simulink model "stpa_brake_manage_loss"  (R2022a)
settings: Solver=VariableStepAuto  StartTime=0.0  StopTime=10.0  RelTol=1e-3
settings Model: Creator=E403510  LastModifiedBy=ayj
settings SolverCC: AlgebraicLoopSolver=TrustRegion
settings DataIOCC: ReturnWorkspaceOutputs=off
settings DebuggingCC: UnconnectedInputMsg=warning  UnconnectedOutputMsg=warning  UnconnectedLineMsg=warning  SFMachineParentedDataDiag=warning  ArithmeticOperatorsInVariantConditions=warning
settings SFSimCC: CustomCodeUndefinedFunction=UseInterfaceOnly

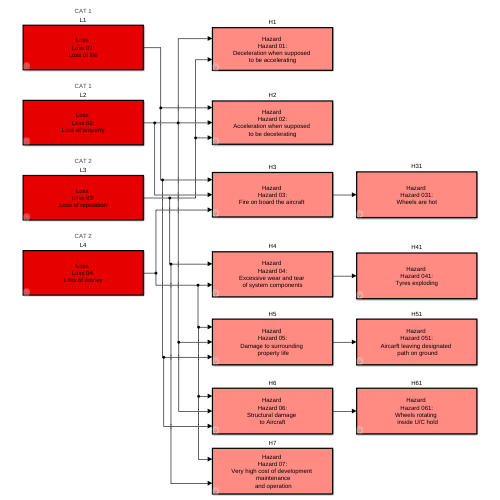
[thumbnail: Simulink's stored preview of the top-level diagram]
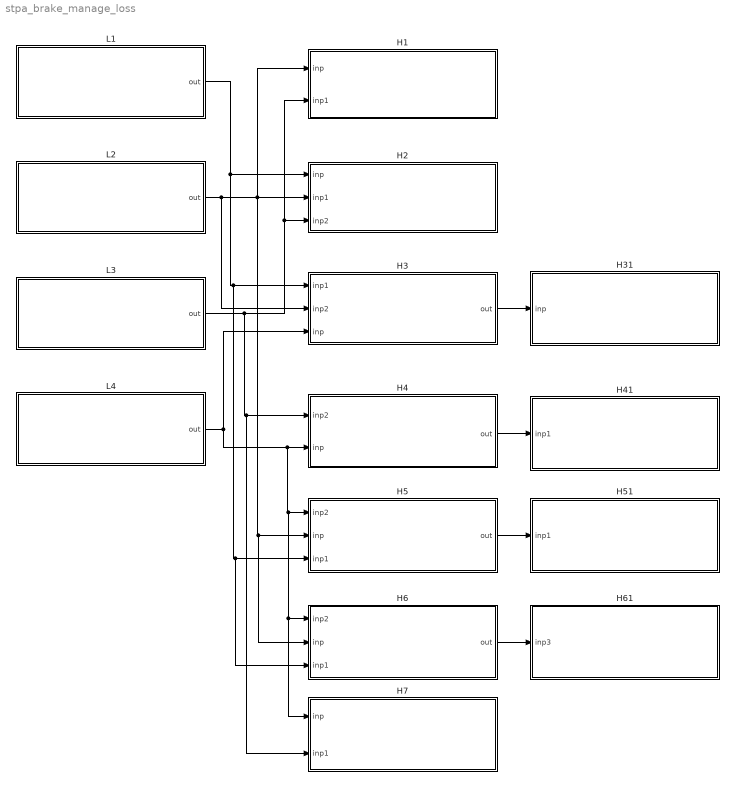
== system stpa_brake_manage_loss ==
  H1 : Subsystem  TreatAsAtomicUnit=on  mask(hazard){NAMEFORBLOCK=Hazard 01, DES=Deceleration when supposed \n to be accelerating}
      mask prompts: NAMEFORBLOCK "Provide a name for Block"; DES "Provide a description of Hazard"
      mask help: Provide details of the Hazard
      mask init:
      | set_param(gcb,'LinkStatus', 'none');
      settings: RTWFcnNameOpts=Use subsystem name  RTWFileNameOpts=Use function name
      mask DialogControl Control2 Prompt: ADD Input
      mask DialogControl Control2 Callback:
      | h = add_block('simulink/Sources/In1', [gcb '/inp'], 'MakeNameUnique', 'on');
      | hg = add_block('simulink/Sinks/Terminator', [gcb '/term'], 'MakeNameUnique', 'on');
      | hname = get_param(h,'PortHandles');
      | hgname = get_param(hg,'PortHandles');
      | add_line(gcb, hname.Outport(1), hgname.Inport(1));
      mask DialogControl Control3 Prompt: ADD Output
      mask DialogControl Control3 Callback:
      | h = add_block('simulink/Sinks/Out1', [gcb '/out'], 'MakeNameUnique', 'on');
      | hg = add_block('simulink/Sources/Ground', [gcb '/gnd'], 'MakeNameUnique', 'on');
      | hname = get_param(h,'PortHandles');
      | hgname = get_param(hg,'PortHandles');
      | add_line(gcb, hgname.Outport(1), hname.Inport(1));
      mask DialogControl Control4 Prompt: REM Input
      mask DialogControl Control4 Callback:
      | a=find_system(gcb,'SearchDepth',2,'LookUnderMasks','all','BlockType','Inport');
      | if ~isempty(a)
      | b=get_param(a{1},'PortConnectivity');
      | delete_block(a{1});
      | delete_block(b.DstBlock);
      | delete_line(find_system(gcb, 'SearchDepth',2,'LookUnderMasks','all','FindAll', 'on', 'Type', 'line', 'Connected', 'off'))
      | end
      mask DialogControl Control5 Prompt: REM Output
      mask DialogControl Control5 Callback:
      | a=find_system(gcb,'SearchDepth',2,'LookUnderMasks','all','BlockType','Outport');
      | if ~isempty(a)
      | b=get_param(a{1},'PortConnectivity');
      | delete_block(a{1});
      | delete_block(b.SrcBlock);
      | delete_line(find_system(gcb, 'SearchDepth',2,'LookUnderMasks','all','FindAll', 'on', 'Type', 'line', 'Connected', 'off'))
      | end
      mask Display: disp(['Hazard \n' NAMEFORBLOCK ':\n' DES])
  H2 : Subsystem  TreatAsAtomicUnit=on  mask(hazard){NAMEFORBLOCK=Hazard 02, DES=Acceleration when supposed \n to be decelerating}
      mask prompts: NAMEFORBLOCK "Provide a name for Block"; DES "Provide a description of Hazard"
      mask help: Provide details of the Hazard
      mask init:
      | set_param(gcb,'LinkStatus', 'none');
      settings: RTWFcnNameOpts=Use subsystem name  RTWFileNameOpts=Use function name
      mask DialogControl Control2 Prompt: ADD Input
      mask DialogControl Control2 Callback:
      | h = add_block('simulink/Sources/In1', [gcb '/inp'], 'MakeNameUnique', 'on');
      | hg = add_block('simulink/Sinks/Terminator', [gcb '/term'], 'MakeNameUnique', 'on');
      | hname = get_param(h,'PortHandles');
      | hgname = get_param(hg,'PortHandles');
      | add_line(gcb, hname.Outport(1), hgname.Inport(1));
      mask DialogControl Control3 Prompt: ADD Output
      mask DialogControl Control3 Callback:
      | h = add_block('simulink/Sinks/Out1', [gcb '/out'], 'MakeNameUnique', 'on');
      | hg = add_block('simulink/Sources/Ground', [gcb '/gnd'], 'MakeNameUnique', 'on');
      | hname = get_param(h,'PortHandles');
      | hgname = get_param(hg,'PortHandles');
      | add_line(gcb, hgname.Outport(1), hname.Inport(1));
      mask DialogControl Control4 Prompt: REM Input
      mask DialogControl Control4 Callback:
      | a=find_system(gcb,'SearchDepth',2,'LookUnderMasks','all','BlockType','Inport');
      | if ~isempty(a)
      | b=get_param(a{1},'PortConnectivity');
      | delete_block(a{1});
      | delete_block(b.DstBlock);
      | delete_line(find_system(gcb, 'SearchDepth',2,'LookUnderMasks','all','FindAll', 'on', 'Type', 'line', 'Connected', 'off'))
      | end
      mask DialogControl Control5 Prompt: REM Output
      mask DialogControl Control5 Callback:
      | a=find_system(gcb,'SearchDepth',2,'LookUnderMasks','all','BlockType','Outport');
      | if ~isempty(a)
      | b=get_param(a{1},'PortConnectivity');
      | delete_block(a{1});
      | delete_block(b.SrcBlock);
      | delete_line(find_system(gcb, 'SearchDepth',2,'LookUnderMasks','all','FindAll', 'on', 'Type', 'line', 'Connected', 'off'))
      | end
      mask Display: disp(['Hazard \n' NAMEFORBLOCK ':\n' DES])
  H3 : Subsystem  TreatAsAtomicUnit=on  mask(hazard){NAMEFORBLOCK=Hazard 03, DES=Fire on board the aircraft}
      mask prompts: NAMEFORBLOCK "Provide a name for Block"; DES "Provide a description of Hazard"
      mask help: Provide details of the Hazard
      mask init:
      | set_param(gcb,'LinkStatus', 'none');
      settings: RTWFcnNameOpts=Use subsystem name  RTWFileNameOpts=Use function name
      mask DialogControl Control2 Prompt: ADD Input
      mask DialogControl Control2 Callback:
      | h = add_block('simulink/Sources/In1', [gcb '/inp'], 'MakeNameUnique', 'on');
      | hg = add_block('simulink/Sinks/Terminator', [gcb '/term'], 'MakeNameUnique', 'on');
      | hname = get_param(h,'PortHandles');
      | hgname = get_param(hg,'PortHandles');
      | add_line(gcb, hname.Outport(1), hgname.Inport(1));
      mask DialogControl Control3 Prompt: ADD Output
      mask DialogControl Control3 Callback:
      | h = add_block('simulink/Sinks/Out1', [gcb '/out'], 'MakeNameUnique', 'on');
      | hg = add_block('simulink/Sources/Ground', [gcb '/gnd'], 'MakeNameUnique', 'on');
      | hname = get_param(h,'PortHandles');
      | hgname = get_param(hg,'PortHandles');
      | add_line(gcb, hgname.Outport(1), hname.Inport(1));
      mask DialogControl Control4 Prompt: REM Input
      mask DialogControl Control4 Callback:
      | a=find_system(gcb,'SearchDepth',2,'LookUnderMasks','all','BlockType','Inport');
      | if ~isempty(a)
      | b=get_param(a{1},'PortConnectivity');
      | delete_block(a{1});
      | delete_block(b.DstBlock);
      | delete_line(find_system(gcb, 'SearchDepth',2,'LookUnderMasks','all','FindAll', 'on', 'Type', 'line', 'Connected', 'off'))
      | end
      mask DialogControl Control5 Prompt: REM Output
      mask DialogControl Control5 Callback:
      | a=find_system(gcb,'SearchDepth',2,'LookUnderMasks','all','BlockType','Outport');
      | if ~isempty(a)
      | b=get_param(a{1},'PortConnectivity');
      | delete_block(a{1});
      | delete_block(b.SrcBlock);
      | delete_line(find_system(gcb, 'SearchDepth',2,'LookUnderMasks','all','FindAll', 'on', 'Type', 'line', 'Connected', 'off'))
      | end
      mask Display: disp(['Hazard \n' NAMEFORBLOCK ':\n' DES])
  H31 : Subsystem  TreatAsAtomicUnit=on  mask(hazard){NAMEFORBLOCK=Hazard 031, DES=Wheels are hot}
      mask prompts: NAMEFORBLOCK "Provide a name for Block"; DES "Provide a description of Hazard"
      mask help: Provide details of the Hazard
      mask init:
      | set_param(gcb,'LinkStatus', 'none');
      settings: RTWFcnNameOpts=Use subsystem name  RTWFileNameOpts=Use function name
      mask DialogControl Control2 Prompt: ADD Input
      mask DialogControl Control2 Callback:
      | h = add_block('simulink/Sources/In1', [gcb '/inp'], 'MakeNameUnique', 'on');
      | hg = add_block('simulink/Sinks/Terminator', [gcb '/term'], 'MakeNameUnique', 'on');
      | hname = get_param(h,'PortHandles');
      | hgname = get_param(hg,'PortHandles');
      | add_line(gcb, hname.Outport(1), hgname.Inport(1));
      mask DialogControl Control3 Prompt: ADD Output
      mask DialogControl Control3 Callback:
      | h = add_block('simulink/Sinks/Out1', [gcb '/out'], 'MakeNameUnique', 'on');
      | hg = add_block('simulink/Sources/Ground', [gcb '/gnd'], 'MakeNameUnique', 'on');
      | hname = get_param(h,'PortHandles');
      | hgname = get_param(hg,'PortHandles');
      | add_line(gcb, hgname.Outport(1), hname.Inport(1));
      mask DialogControl Control4 Prompt: REM Input
      mask DialogControl Control4 Callback:
      | a=find_system(gcb,'SearchDepth',2,'LookUnderMasks','all','BlockType','Inport');
      | if ~isempty(a)
      | b=get_param(a{1},'PortConnectivity');
      | delete_block(a{1});
      | delete_block(b.DstBlock);
      | delete_line(find_system(gcb, 'SearchDepth',2,'LookUnderMasks','all','FindAll', 'on', 'Type', 'line', 'Connected', 'off'))
      | end
      mask DialogControl Control5 Prompt: REM Output
      mask DialogControl Control5 Callback:
      | a=find_system(gcb,'SearchDepth',2,'LookUnderMasks','all','BlockType','Outport');
      | if ~isempty(a)
      | b=get_param(a{1},'PortConnectivity');
      | delete_block(a{1});
      | delete_block(b.SrcBlock);
      | delete_line(find_system(gcb, 'SearchDepth',2,'LookUnderMasks','all','FindAll', 'on', 'Type', 'line', 'Connected', 'off'))
      | end
      mask Display: disp(['Hazard \n' NAMEFORBLOCK ':\n' DES])
  H4 : Subsystem  TreatAsAtomicUnit=on  mask(hazard){NAMEFORBLOCK=Hazard 04, DES=Excessive wear and tear \n of system components}
      mask prompts: NAMEFORBLOCK "Provide a name for Block"; DES "Provide a description of Hazard"
      mask help: Provide details of the Hazard
      mask init:
      | set_param(gcb,'LinkStatus', 'none');
      settings: RTWFcnNameOpts=Use subsystem name  RTWFileNameOpts=Use function name
      mask DialogControl Control2 Prompt: ADD Input
      mask DialogControl Control2 Callback:
      | h = add_block('simulink/Sources/In1', [gcb '/inp'], 'MakeNameUnique', 'on');
      | hg = add_block('simulink/Sinks/Terminator', [gcb '/term'], 'MakeNameUnique', 'on');
      | hname = get_param(h,'PortHandles');
      | hgname = get_param(hg,'PortHandles');
      | add_line(gcb, hname.Outport(1), hgname.Inport(1));
      mask DialogControl Control3 Prompt: ADD Output
      mask DialogControl Control3 Callback:
      | h = add_block('simulink/Sinks/Out1', [gcb '/out'], 'MakeNameUnique', 'on');
      | hg = add_block('simulink/Sources/Ground', [gcb '/gnd'], 'MakeNameUnique', 'on');
      | hname = get_param(h,'PortHandles');
      | hgname = get_param(hg,'PortHandles');
      | add_line(gcb, hgname.Outport(1), hname.Inport(1));
      mask DialogControl Control4 Prompt: REM Input
      mask DialogControl Control4 Callback:
      | a=find_system(gcb,'SearchDepth',2,'LookUnderMasks','all','BlockType','Inport');
      | if ~isempty(a)
      | b=get_param(a{1},'PortConnectivity');
      | delete_block(a{1});
      | delete_block(b.DstBlock);
      | delete_line(find_system(gcb, 'SearchDepth',2,'LookUnderMasks','all','FindAll', 'on', 'Type', 'line', 'Connected', 'off'))
      | end
      mask DialogControl Control5 Prompt: REM Output
      mask DialogControl Control5 Callback:
      | a=find_system(gcb,'SearchDepth',2,'LookUnderMasks','all','BlockType','Outport');
      | if ~isempty(a)
      | b=get_param(a{1},'PortConnectivity');
      | delete_block(a{1});
      | delete_block(b.SrcBlock);
      | delete_line(find_system(gcb, 'SearchDepth',2,'LookUnderMasks','all','FindAll', 'on', 'Type', 'line', 'Connected', 'off'))
      | end
      mask Display: disp(['Hazard \n' NAMEFORBLOCK ':\n' DES])
  H41 : Subsystem  TreatAsAtomicUnit=on  mask(hazard){NAMEFORBLOCK=Hazard 041, DES=Tyres exploding}
      mask prompts: NAMEFORBLOCK "Provide a name for Block"; DES "Provide a description of Hazard"
      mask help: Provide details of the Hazard
      mask init:
      | set_param(gcb,'LinkStatus', 'none');
      settings: RTWFcnNameOpts=Use subsystem name  RTWFileNameOpts=Use function name
      mask DialogControl Control2 Prompt: ADD Input
      mask DialogControl Control2 Callback:
      | h = add_block('simulink/Sources/In1', [gcb '/inp'], 'MakeNameUnique', 'on');
      | hg = add_block('simulink/Sinks/Terminator', [gcb '/term'], 'MakeNameUnique', 'on');
      | hname = get_param(h,'PortHandles');
      | hgname = get_param(hg,'PortHandles');
      | add_line(gcb, hname.Outport(1), hgname.Inport(1));
      mask DialogControl Control3 Prompt: ADD Output
      mask DialogControl Control3 Callback:
      | h = add_block('simulink/Sinks/Out1', [gcb '/out'], 'MakeNameUnique', 'on');
      | hg = add_block('simulink/Sources/Ground', [gcb '/gnd'], 'MakeNameUnique', 'on');
      | hname = get_param(h,'PortHandles');
      | hgname = get_param(hg,'PortHandles');
      | add_line(gcb, hgname.Outport(1), hname.Inport(1));
      mask DialogControl Control4 Prompt: REM Input
      mask DialogControl Control4 Callback:
      | a=find_system(gcb,'SearchDepth',2,'LookUnderMasks','all','BlockType','Inport');
      | if ~isempty(a)
      | b=get_param(a{1},'PortConnectivity');
      | delete_block(a{1});
      | delete_block(b.DstBlock);
      | delete_line(find_system(gcb, 'SearchDepth',2,'LookUnderMasks','all','FindAll', 'on', 'Type', 'line', 'Connected', 'off'))
      | end
      mask DialogControl Control5 Prompt: REM Output
      mask DialogControl Control5 Callback:
      | a=find_system(gcb,'SearchDepth',2,'LookUnderMasks','all','BlockType','Outport');
      | if ~isempty(a)
      | b=get_param(a{1},'PortConnectivity');
      | delete_block(a{1});
      | delete_block(b.SrcBlock);
      | delete_line(find_system(gcb, 'SearchDepth',2,'LookUnderMasks','all','FindAll', 'on', 'Type', 'line', 'Connected', 'off'))
      | end
      mask Display: disp(['Hazard \n' NAMEFORBLOCK ':\n' DES])
  H5 : Subsystem  TreatAsAtomicUnit=on  mask(hazard){NAMEFORBLOCK=Hazard 05, DES=Damage to surrounding \n property life}
      mask prompts: NAMEFORBLOCK "Provide a name for Block"; DES "Provide a description of Hazard"
      mask help: Provide details of the Hazard
      mask init:
      | set_param(gcb,'LinkStatus', 'none');
      settings: RTWFcnNameOpts=Use subsystem name  RTWFileNameOpts=Use function name
      mask DialogControl Control2 Prompt: ADD Input
      mask DialogControl Control2 Callback:
      | h = add_block('simulink/Sources/In1', [gcb '/inp'], 'MakeNameUnique', 'on');
      | hg = add_block('simulink/Sinks/Terminator', [gcb '/term'], 'MakeNameUnique', 'on');
      | hname = get_param(h,'PortHandles');
      | hgname = get_param(hg,'PortHandles');
      | add_line(gcb, hname.Outport(1), hgname.Inport(1));
      mask DialogControl Control3 Prompt: ADD Output
      mask DialogControl Control3 Callback:
      | h = add_block('simulink/Sinks/Out1', [gcb '/out'], 'MakeNameUnique', 'on');
      | hg = add_block('simulink/Sources/Ground', [gcb '/gnd'], 'MakeNameUnique', 'on');
      | hname = get_param(h,'PortHandles');
      | hgname = get_param(hg,'PortHandles');
      | add_line(gcb, hgname.Outport(1), hname.Inport(1));
      mask DialogControl Control4 Prompt: REM Input
      mask DialogControl Control4 Callback:
      | a=find_system(gcb,'SearchDepth',2,'LookUnderMasks','all','BlockType','Inport');
      | if ~isempty(a)
      | b=get_param(a{1},'PortConnectivity');
      | delete_block(a{1});
      | delete_block(b.DstBlock);
      | delete_line(find_system(gcb, 'SearchDepth',2,'LookUnderMasks','all','FindAll', 'on', 'Type', 'line', 'Connected', 'off'))
      | end
      mask DialogControl Control5 Prompt: REM Output
      mask DialogControl Control5 Callback:
      | a=find_system(gcb,'SearchDepth',2,'LookUnderMasks','all','BlockType','Outport');
      | if ~isempty(a)
      | b=get_param(a{1},'PortConnectivity');
      | delete_block(a{1});
      | delete_block(b.SrcBlock);
      | delete_line(find_system(gcb, 'SearchDepth',2,'LookUnderMasks','all','FindAll', 'on', 'Type', 'line', 'Connected', 'off'))
      | end
      mask Display: disp(['Hazard \n' NAMEFORBLOCK ':\n' DES])
  H51 : Subsystem  TreatAsAtomicUnit=on  mask(hazard){NAMEFORBLOCK=Hazard 051, DES=Aircarft leaving designated \n path on ground}
      mask prompts: NAMEFORBLOCK "Provide a name for Block"; DES "Provide a description of Hazard"
      mask help: Provide details of the Hazard
      mask init:
      | set_param(gcb,'LinkStatus', 'none');
      settings: RTWFcnNameOpts=Use subsystem name  RTWFileNameOpts=Use function name
      mask DialogControl Control2 Prompt: ADD Input
      mask DialogControl Control2 Callback:
      | h = add_block('simulink/Sources/In1', [gcb '/inp'], 'MakeNameUnique', 'on');
      | hg = add_block('simulink/Sinks/Terminator', [gcb '/term'], 'MakeNameUnique', 'on');
      | hname = get_param(h,'PortHandles');
      | hgname = get_param(hg,'PortHandles');
      | add_line(gcb, hname.Outport(1), hgname.Inport(1));
      mask DialogControl Control3 Prompt: ADD Output
      mask DialogControl Control3 Callback:
      | h = add_block('simulink/Sinks/Out1', [gcb '/out'], 'MakeNameUnique', 'on');
      | hg = add_block('simulink/Sources/Ground', [gcb '/gnd'], 'MakeNameUnique', 'on');
      | hname = get_param(h,'PortHandles');
      | hgname = get_param(hg,'PortHandles');
      | add_line(gcb, hgname.Outport(1), hname.Inport(1));
      mask DialogControl Control4 Prompt: REM Input
      mask DialogControl Control4 Callback:
      | a=find_system(gcb,'SearchDepth',2,'LookUnderMasks','all','BlockType','Inport');
      | if ~isempty(a)
      | b=get_param(a{1},'PortConnectivity');
      | delete_block(a{1});
      | delete_block(b.DstBlock);
      | delete_line(find_system(gcb, 'SearchDepth',2,'LookUnderMasks','all','FindAll', 'on', 'Type', 'line', 'Connected', 'off'))
      | end
      mask DialogControl Control5 Prompt: REM Output
      mask DialogControl Control5 Callback:
      | a=find_system(gcb,'SearchDepth',2,'LookUnderMasks','all','BlockType','Outport');
      | if ~isempty(a)
      | b=get_param(a{1},'PortConnectivity');
      | delete_block(a{1});
      | delete_block(b.SrcBlock);
      | delete_line(find_system(gcb, 'SearchDepth',2,'LookUnderMasks','all','FindAll', 'on', 'Type', 'line', 'Connected', 'off'))
      | end
      mask Display: disp(['Hazard \n' NAMEFORBLOCK ':\n' DES])
  H6 : Subsystem  TreatAsAtomicUnit=on  mask(hazard){NAMEFORBLOCK=Hazard 06, DES=Structural damage \n to Aircraft}
      mask prompts: NAMEFORBLOCK "Provide a name for Block"; DES "Provide a description of Hazard"
      mask help: Provide details of the Hazard
      mask init:
      | set_param(gcb,'LinkStatus', 'none');
      settings: RTWFcnNameOpts=Use subsystem name  RTWFileNameOpts=Use function name
      mask DialogControl Control2 Prompt: ADD Input
      mask DialogControl Control2 Callback:
      | h = add_block('simulink/Sources/In1', [gcb '/inp'], 'MakeNameUnique', 'on');
      | hg = add_block('simulink/Sinks/Terminator', [gcb '/term'], 'MakeNameUnique', 'on');
      | hname = get_param(h,'PortHandles');
      | hgname = get_param(hg,'PortHandles');
      | add_line(gcb, hname.Outport(1), hgname.Inport(1));
      mask DialogControl Control3 Prompt: ADD Output
      mask DialogControl Control3 Callback:
      | h = add_block('simulink/Sinks/Out1', [gcb '/out'], 'MakeNameUnique', 'on');
      | hg = add_block('simulink/Sources/Ground', [gcb '/gnd'], 'MakeNameUnique', 'on');
      | hname = get_param(h,'PortHandles');
      | hgname = get_param(hg,'PortHandles');
      | add_line(gcb, hgname.Outport(1), hname.Inport(1));
      mask DialogControl Control4 Prompt: REM Input
      mask DialogControl Control4 Callback:
      | a=find_system(gcb,'SearchDepth',2,'LookUnderMasks','all','BlockType','Inport');
      | if ~isempty(a)
      | b=get_param(a{1},'PortConnectivity');
      | delete_block(a{1});
      | delete_block(b.DstBlock);
      | delete_line(find_system(gcb, 'SearchDepth',2,'LookUnderMasks','all','FindAll', 'on', 'Type', 'line', 'Connected', 'off'))
      | end
      mask DialogControl Control5 Prompt: REM Output
      mask DialogControl Control5 Callback:
      | a=find_system(gcb,'SearchDepth',2,'LookUnderMasks','all','BlockType','Outport');
      | if ~isempty(a)
      | b=get_param(a{1},'PortConnectivity');
      | delete_block(a{1});
      | delete_block(b.SrcBlock);
      | delete_line(find_system(gcb, 'SearchDepth',2,'LookUnderMasks','all','FindAll', 'on', 'Type', 'line', 'Connected', 'off'))
      | end
      mask Display: disp(['Hazard \n' NAMEFORBLOCK ':\n' DES])
  H61 : Subsystem  TreatAsAtomicUnit=on  mask(hazard){NAMEFORBLOCK=Hazard 061, DES=Wheels rotating \n inside U/C hold}
      mask prompts: NAMEFORBLOCK "Provide a name for Block"; DES "Provide a description of Hazard"
      mask help: Provide details of the Hazard
      mask init:
      | set_param(gcb,'LinkStatus', 'none');
      settings: RTWFcnNameOpts=Use subsystem name  RTWFileNameOpts=Use function name
      mask DialogControl Control2 Prompt: ADD Input
      mask DialogControl Control2 Callback:
      | h = add_block('simulink/Sources/In1', [gcb '/inp'], 'MakeNameUnique', 'on');
      | hg = add_block('simulink/Sinks/Terminator', [gcb '/term'], 'MakeNameUnique', 'on');
      | hname = get_param(h,'PortHandles');
      | hgname = get_param(hg,'PortHandles');
      | add_line(gcb, hname.Outport(1), hgname.Inport(1));
      mask DialogControl Control3 Prompt: ADD Output
      mask DialogControl Control3 Callback:
      | h = add_block('simulink/Sinks/Out1', [gcb '/out'], 'MakeNameUnique', 'on');
      | hg = add_block('simulink/Sources/Ground', [gcb '/gnd'], 'MakeNameUnique', 'on');
      | hname = get_param(h,'PortHandles');
      | hgname = get_param(hg,'PortHandles');
      | add_line(gcb, hgname.Outport(1), hname.Inport(1));
      mask DialogControl Control4 Prompt: REM Input
      mask DialogControl Control4 Callback:
      | a=find_system(gcb,'SearchDepth',2,'LookUnderMasks','all','BlockType','Inport');
      | if ~isempty(a)
      | b=get_param(a{1},'PortConnectivity');
      | delete_block(a{1});
      | delete_block(b.DstBlock);
      | delete_line(find_system(gcb, 'SearchDepth',2,'LookUnderMasks','all','FindAll', 'on', 'Type', 'line', 'Connected', 'off'))
      | end
      mask DialogControl Control5 Prompt: REM Output
      mask DialogControl Control5 Callback:
      | a=find_system(gcb,'SearchDepth',2,'LookUnderMasks','all','BlockType','Outport');
      | if ~isempty(a)
      | b=get_param(a{1},'PortConnectivity');
      | delete_block(a{1});
      | delete_block(b.SrcBlock);
      | delete_line(find_system(gcb, 'SearchDepth',2,'LookUnderMasks','all','FindAll', 'on', 'Type', 'line', 'Connected', 'off'))
      | end
      mask Display: disp(['Hazard \n' NAMEFORBLOCK ':\n' DES])
  H7 : Subsystem  TreatAsAtomicUnit=on  mask(hazard){NAMEFORBLOCK=Hazard 07, DES=Very high cost of development \n maintenance\n and operation}
      mask prompts: NAMEFORBLOCK "Provide a name for Block"; DES "Provide a description of Hazard"
      mask help: Provide details of the Hazard
      mask init:
      | set_param(gcb,'LinkStatus', 'none');
      settings: RTWFcnNameOpts=Use subsystem name  RTWFileNameOpts=Use function name
      mask DialogControl Control2 Prompt: ADD Input
      mask DialogControl Control2 Callback:
      | h = add_block('simulink/Sources/In1', [gcb '/inp'], 'MakeNameUnique', 'on');
      | hg = add_block('simulink/Sinks/Terminator', [gcb '/term'], 'MakeNameUnique', 'on');
      | hname = get_param(h,'PortHandles');
      | hgname = get_param(hg,'PortHandles');
      | add_line(gcb, hname.Outport(1), hgname.Inport(1));
      mask DialogControl Control3 Prompt: ADD Output
      mask DialogControl Control3 Callback:
      | h = add_block('simulink/Sinks/Out1', [gcb '/out'], 'MakeNameUnique', 'on');
      | hg = add_block('simulink/Sources/Ground', [gcb '/gnd'], 'MakeNameUnique', 'on');
      | hname = get_param(h,'PortHandles');
      | hgname = get_param(hg,'PortHandles');
      | add_line(gcb, hgname.Outport(1), hname.Inport(1));
      mask DialogControl Control4 Prompt: REM Input
      mask DialogControl Control4 Callback:
      | a=find_system(gcb,'SearchDepth',2,'LookUnderMasks','all','BlockType','Inport');
      | if ~isempty(a)
      | b=get_param(a{1},'PortConnectivity');
      | delete_block(a{1});
      | delete_block(b.DstBlock);
      | delete_line(find_system(gcb, 'SearchDepth',2,'LookUnderMasks','all','FindAll', 'on', 'Type', 'line', 'Connected', 'off'))
      | end
      mask DialogControl Control5 Prompt: REM Output
      mask DialogControl Control5 Callback:
      | a=find_system(gcb,'SearchDepth',2,'LookUnderMasks','all','BlockType','Outport');
      | if ~isempty(a)
      | b=get_param(a{1},'PortConnectivity');
      | delete_block(a{1});
      | delete_block(b.SrcBlock);
      | delete_line(find_system(gcb, 'SearchDepth',2,'LookUnderMasks','all','FindAll', 'on', 'Type', 'line', 'Connected', 'off'))
      | end
      mask Display: disp(['Hazard \n' NAMEFORBLOCK ':\n' DES])
  L1 : Subsystem  TreatAsAtomicUnit=on  mask(loss){NAMEFORBLOCK=Loss 01, DES=Loss of life, LOSSCAT=1}
      mask prompts: NAMEFORBLOCK "Provide a name for Block"; DES "Provide a description of Loss"; LOSSCAT "Provide Loss Category CAT 1, 2, 3"
      mask help: Provide details of the loss
      mask init:
      | set_param(gcb,'LinkStatus', 'none');
      settings: AttributesFormatString=CAT %<LOSSCAT>  RTWFcnNameOpts=Use subsystem name  RTWFileNameOpts=Use function name
      mask DialogControl Control3 Prompt: ADD Output
      mask DialogControl Control3 Callback:
      | h = add_block('simulink/Sinks/Out1', [gcb '/out'], 'MakeNameUnique', 'on');
      | hg = add_block('simulink/Sources/Ground', [gcb '/gnd'], 'MakeNameUnique', 'on');
      | hname = get_param(h,'PortHandles');
      | hgname = get_param(hg,'PortHandles');
      | add_line(gcb, hgname.Outport(1), hname.Inport(1));
      mask DialogControl Control5 Prompt: REM Output
      mask DialogControl Control5 Callback:
      | a=find_system(gcb,'SearchDepth',2,'LookUnderMasks','all','BlockType','Outport');
      | if ~isempty(a)
      | b=get_param(a{1},'PortConnectivity');
      | delete_block(a{1});
      | delete_block(b.SrcBlock);
      | delete_line(find_system(gcb, 'SearchDepth',2,'LookUnderMasks','all','FindAll', 'on', 'Type', 'line', 'Connected', 'off'))
      | end
      mask Display: disp(['Loss \n' NAMEFORBLOCK ':\n' DES])
  L2 : Subsystem  TreatAsAtomicUnit=on  mask(loss){NAMEFORBLOCK=Loss 02, DES=Loss of property, LOSSCAT=1}
      mask prompts: NAMEFORBLOCK "Provide a name for Block"; DES "Provide a description of Loss"; LOSSCAT "Provide Loss Category CAT 1, 2, 3"
      mask help: Provide details of the loss
      mask init:
      | set_param(gcb,'LinkStatus', 'none');
      settings: AttributesFormatString=CAT %<LOSSCAT>  RTWFcnNameOpts=Use subsystem name  RTWFileNameOpts=Use function name
      mask DialogControl Control3 Prompt: ADD Output
      mask DialogControl Control3 Callback:
      | h = add_block('simulink/Sinks/Out1', [gcb '/out'], 'MakeNameUnique', 'on');
      | hg = add_block('simulink/Sources/Ground', [gcb '/gnd'], 'MakeNameUnique', 'on');
      | hname = get_param(h,'PortHandles');
      | hgname = get_param(hg,'PortHandles');
      | add_line(gcb, hgname.Outport(1), hname.Inport(1));
      mask DialogControl Control5 Prompt: REM Output
      mask DialogControl Control5 Callback:
      | a=find_system(gcb,'SearchDepth',2,'LookUnderMasks','all','BlockType','Outport');
      | if ~isempty(a)
      | b=get_param(a{1},'PortConnectivity');
      | delete_block(a{1});
      | delete_block(b.SrcBlock);
      | delete_line(find_system(gcb, 'SearchDepth',2,'LookUnderMasks','all','FindAll', 'on', 'Type', 'line', 'Connected', 'off'))
      | end
      mask Display: disp(['Loss \n' NAMEFORBLOCK ':\n' DES])
  L3 : Subsystem  TreatAsAtomicUnit=on  mask(loss){NAMEFORBLOCK=Loss 03, DES=Loss of reputation, LOSSCAT=2}
      mask prompts: NAMEFORBLOCK "Provide a name for Block"; DES "Provide a description of Loss"; LOSSCAT "Provide Loss Category CAT 1, 2, 3"
      mask help: Provide details of the loss
      mask init:
      | set_param(gcb,'LinkStatus', 'none');
      settings: AttributesFormatString=CAT %<LOSSCAT>  RTWFcnNameOpts=Use subsystem name  RTWFileNameOpts=Use function name
      mask DialogControl Control3 Prompt: ADD Output
      mask DialogControl Control3 Callback:
      | h = add_block('simulink/Sinks/Out1', [gcb '/out'], 'MakeNameUnique', 'on');
      | hg = add_block('simulink/Sources/Ground', [gcb '/gnd'], 'MakeNameUnique', 'on');
      | hname = get_param(h,'PortHandles');
      | hgname = get_param(hg,'PortHandles');
      | add_line(gcb, hgname.Outport(1), hname.Inport(1));
      mask DialogControl Control5 Prompt: REM Output
      mask DialogControl Control5 Callback:
      | a=find_system(gcb,'SearchDepth',2,'LookUnderMasks','all','BlockType','Outport');
      | if ~isempty(a)
      | b=get_param(a{1},'PortConnectivity');
      | delete_block(a{1});
      | delete_block(b.SrcBlock);
      | delete_line(find_system(gcb, 'SearchDepth',2,'LookUnderMasks','all','FindAll', 'on', 'Type', 'line', 'Connected', 'off'))
      | end
      mask Display: disp(['Loss \n' NAMEFORBLOCK ':\n' DES])
  L4 : Subsystem  TreatAsAtomicUnit=on  mask(loss){NAMEFORBLOCK=Loss 04, DES=Loss of money, LOSSCAT=2}
      mask prompts: NAMEFORBLOCK "Provide a name for Block"; DES "Provide a description of Loss"; LOSSCAT "Provide Loss Category CAT 1, 2, 3"
      mask help: Provide details of the loss
      mask init:
      | set_param(gcb,'LinkStatus', 'none');
      settings: AttributesFormatString=CAT %<LOSSCAT>  RTWFcnNameOpts=Use subsystem name  RTWFileNameOpts=Use function name
      mask DialogControl Control3 Prompt: ADD Output
      mask DialogControl Control3 Callback:
      | h = add_block('simulink/Sinks/Out1', [gcb '/out'], 'MakeNameUnique', 'on');
      | hg = add_block('simulink/Sources/Ground', [gcb '/gnd'], 'MakeNameUnique', 'on');
      | hname = get_param(h,'PortHandles');
      | hgname = get_param(hg,'PortHandles');
      | add_line(gcb, hgname.Outport(1), hname.Inport(1));
      mask DialogControl Control5 Prompt: REM Output
      mask DialogControl Control5 Callback:
      | a=find_system(gcb,'SearchDepth',2,'LookUnderMasks','all','BlockType','Outport');
      | if ~isempty(a)
      | b=get_param(a{1},'PortConnectivity');
      | delete_block(a{1});
      | delete_block(b.SrcBlock);
      | delete_line(find_system(gcb, 'SearchDepth',2,'LookUnderMasks','all','FindAll', 'on', 'Type', 'line', 'Connected', 'off'))
      | end
      mask Display: disp(['Loss \n' NAMEFORBLOCK ':\n' DES])
  wires:
  L2/1(out) -> H3/2(inp2), H6/2(inp), H5/2(inp), H2/2(inp1), H1/1(inp)
  L3/1(out) -> H7/2(inp1), H4/1(inp2), H2/3(inp2), H1/2(inp1)
  L1/1(out) -> H2/1(inp), H6/3(inp1), H5/3(inp1), H3/1(inp1)
  L4/1(out) -> H6/1(inp2), H7/1(inp), H5/1(inp2), H4/2(inp), H3/3(inp)
  H3/1(out) -> H31/1(inp)
  H6/1(out) -> H61/1(inp3)
  H5/1(out) -> H51/1(inp1)
  H4/1(out) -> H41/1(inp1)

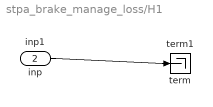
== system stpa_brake_manage_loss/H1 ==
  inp : Inport
  inp1 : Inport  Port=2
  term : Terminator
  term1 : Terminator
  wires:
  inp/1 -> term/1
  inp1/1 -> term1/1

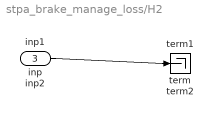
== system stpa_brake_manage_loss/H2 ==
  inp : Inport
  inp1 : Inport  Port=2
  inp2 : Inport  Port=3
  term : Terminator
  term1 : Terminator
  term2 : Terminator
  wires:
  inp1/1 -> term1/1
  inp/1 -> term/1
  inp2/1 -> term2/1

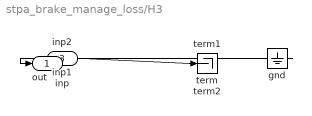
== system stpa_brake_manage_loss/H3 ==
  inp1 : Inport
  inp2 : Inport  Port=2
  inp : Inport  Port=3
  gnd : Ground
  term : Terminator
  term1 : Terminator
  term2 : Terminator
  out : Outport  VectorParamsAs1DForOutWhenUnconnected=off
  wires:
  inp2/1 -> term2/1
  inp1/1 -> term1/1
  inp/1 -> term/1
  gnd/1 -> out/1

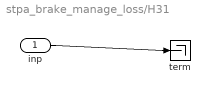
== system stpa_brake_manage_loss/H31 ==
  inp : Inport
  term : Terminator
  wires:
  inp/1 -> term/1

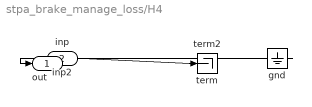
== system stpa_brake_manage_loss/H4 ==
  inp2 : Inport
  inp : Inport  Port=2
  gnd : Ground
  term : Terminator
  term2 : Terminator
  out : Outport
  wires:
  inp/1 -> term/1
  inp2/1 -> term2/1
  gnd/1 -> out/1

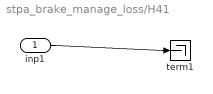
== system stpa_brake_manage_loss/H41 ==
  inp1 : Inport
  term1 : Terminator
  wires:
  inp1/1 -> term1/1

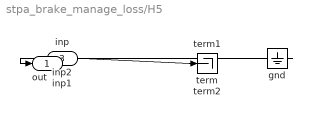
== system stpa_brake_manage_loss/H5 ==
  inp2 : Inport
  inp : Inport  Port=2
  inp1 : Inport  Port=3
  gnd : Ground
  term : Terminator
  term1 : Terminator
  term2 : Terminator
  out : Outport
  wires:
  inp2/1 -> term2/1
  inp/1 -> term/1
  inp1/1 -> term1/1
  gnd/1 -> out/1

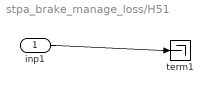
== system stpa_brake_manage_loss/H51 ==
  inp1 : Inport
  term1 : Terminator
  wires:
  inp1/1 -> term1/1

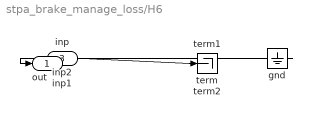
== system stpa_brake_manage_loss/H6 ==
  inp2 : Inport
  inp : Inport  Port=2
  inp1 : Inport  Port=3
  gnd : Ground
  term : Terminator
  term1 : Terminator
  term2 : Terminator
  out : Outport
  wires:
  inp1/1 -> term1/1
  inp/1 -> term/1
  inp2/1 -> term2/1
  gnd/1 -> out/1

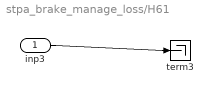
== system stpa_brake_manage_loss/H61 ==
  inp3 : Inport
  term3 : Terminator
  wires:
  inp3/1 -> term3/1

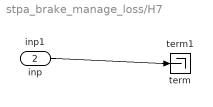
== system stpa_brake_manage_loss/H7 ==
  inp : Inport
  inp1 : Inport  Port=2
  term : Terminator
  term1 : Terminator
  wires:
  inp/1 -> term/1
  inp1/1 -> term1/1

== system stpa_brake_manage_loss/L1 ==
  gnd : Ground
  out : Outport  VectorParamsAs1DForOutWhenUnconnected=off
  wires:
  gnd/1 -> out/1

== system stpa_brake_manage_loss/L2 ==
  gnd : Ground
  out : Outport  VectorParamsAs1DForOutWhenUnconnected=off
  wires:
  gnd/1 -> out/1

== system stpa_brake_manage_loss/L3 ==
  gnd : Ground
  out : Outport  VectorParamsAs1DForOutWhenUnconnected=off
  wires:
  gnd/1 -> out/1

== system stpa_brake_manage_loss/L4 ==
  gnd : Ground
  out : Outport  VectorParamsAs1DForOutWhenUnconnected=off
  wires:
  gnd/1 -> out/1
